simulink model "KiemnghiemDatathudc"  (R2021b)
settings: Solver=VariableStepAuto  StartTime=0.0  StopTime=10  RelTol=1e-3
InitFcn:
  | x_ref = 1; l_ref =0.2; l_ini = 0.6;
  | 
  | %ADRC' s parameter caculation
  | b0 = (ml+mc)/(mc*ml +mc*mt+ml*mt);k_ESO = 70;T_set  = 3;
  | 
  | s_cl = -5.85/T_set;
  | Kp   = s_cl^2;
  | Kd   = -2*s_cl;
  | 
  | s_ESO = k_ESO*s_cl;
  | l1        = -3*s_ESO;
  | l2        = 3*( s_ESO)^2;
  | l3        = -(s_ESO)^3;
  | 
  | %Observer
  | A = [-l1, 1, 0;
  |         -l2, 0, 1;
  |         -l3, 0, 0];
  | B = [0;
  |         b0;
  |         0];
  | L = [l1;
  |        l2;
  |        l3];
  | 
  | b1 = (mt+mc)/(mc*ml +mc*mt+ml*mt);k_ESO1 =100;T_set1  = 3;
  | s_cl1 = -5.85/T_set1;
  | Kp1   = s_cl1^2;
  | Kd1   = -2*s_cl1;
  | 
  | s_ESO1 = k_ESO1*s_cl1;
  | l11        = -3*s_ESO1;
  | l21        = 3*( s_ESO1)^2;
  | l31        = -(s_ESO1)^3;
  | 
  | %Observer
  | A1 = [-l11, 1, 0;
  |         -l21, 0, 1;
  |         -l31, 0, 0];
  | B1 = [0;
  |         b1;
  |         0];
  | L1 = [l11;
  |        l21;
  |        l31];
values from neighbouring files (symbols this model uses):
  g = 9.81    [Thong_so_double_pendulum.m]
undefined symbols (not defined in the file or in its folder): K_pso, mc, sigbuilder_block, T_pso, waof, waol
libraries: neural x95, simulink x11, simulink_extras x11
(part 2 of 6)

== system KiemnghiemDatathudc/data_l_conzvd_3neuron/Custom Neural Network ==
  Input : Inport  PortDimensions=1
      mask Display: e = 0.06;c1 = [120 230 180]/255;c2 = ([120 230 180]+0)/(256+128);c3 = ([120 230 180]+128)/(256+128);patch([0 1 1 0],[0 0 1 1],c1);patch([0 1 1 1-e 1-e 0+e],[0 0 1 1-e 0+e 0+e],c2);patch([0 0 1 1-e 0+e 0+e],[0 1 1 1-e 1-e 0+e],c3);plot([0 1 1 0 0],[0 0 1 1 0]);
  Layer 1 : Subsystem
      mask Display: e = 0.06;c1 = [120 150 230]/255;c2 = ([120 150 230]+0)/383;c3 = ([120 150 230]+128)/383;patch([0 1 1 0],[0 0 1 1],c1);patch([0 1 1 1-e 1-e 0+e],[0 0 1 1-e 0+e 0+e],c2);patch([0 0 1 1-e 0+e 0+e],[0 1 1 1-e 1-e 0+e],c3);plot([0 1 1 0 0],[0 0 1 1 0]);
  Layer 2 : Subsystem
      mask Display: e = 0.06;c1 = [120 150 230]/255;c2 = ([120 150 230]+0)/383;c3 = ([120 150 230]+128)/383;patch([0 1 1 0],[0 0 1 1],c1);patch([0 1 1 1-e 1-e 0+e],[0 0 1 1-e 0+e 0+e],c2);patch([0 0 1 1-e 0+e 0+e],[0 1 1 1-e 1-e 0+e],c3);plot([0 1 1 0 0],[0 0 1 1 0]);
  Process Input 1 : Subsystem
      mask Display: e = 0.06;c1 = [120 150 230]/255;c2 = ([120 150 230]+0)/383;c3 = ([120 150 230]+128)/383;patch([0 1 1 0],[0 0 1 1],c1);patch([0 1 1 1-e 1-e 0+e],[0 0 1 1-e 0+e 0+e],c2);patch([0 0 1 1-e 0+e 0+e],[0 1 1 1-e 1-e 0+e],c3);plot([0 1 1 0 0],[0 0 1 1 0]);
  Process Output 1 : Subsystem
      mask Display: e = 0.06;c1 = [120 150 230]/255;c2 = ([120 150 230]+0)/383;c3 = ([120 150 230]+128)/383;patch([0 1 1 0],[0 0 1 1],c1);patch([0 1 1 1-e 1-e 0+e],[0 0 1 1-e 0+e 0+e],c2);patch([0 0 1 1-e 0+e 0+e],[0 1 1 1-e 1-e 0+e],c3);plot([0 1 1 0 0],[0 0 1 1 0]);
  Output : Outport  InitialOutput=[0;0]
      mask Display: e = 0.06;c1 = [120 230 180]/255;c2 = ([120 230 180]+0)/(256+128);c3 = ([120 230 180]+128)/(256+128);patch([0 1 1 0],[0 0 1 1],c1);patch([0 1 1 1-e 1-e 0+e],[0 0 1 1-e 0+e 0+e],c2);patch([0 0 1 1-e 0+e 0+e],[0 1 1 1-e 1-e 0+e],c3);plot([0 1 1 0 0],[0 0 1 1 0]);
  wires:
  Input/1 -> Process Input 1/1(x)
  Process Output 1/1(y) -> Output/1
  Process Input 1/1(p) -> Layer 1/1("p{1}")
  Layer 1/1("a{1}") -> [feedback1]
  [feedback1] -> Layer 2/1("a{1} ")
  Layer 2/1("a{2}") -> Process Output 1/1(a)

== system KiemnghiemDatathudc/data_l_conzvd_3neuron/Fitness APS ZVD4 ==
  e : Inport
  Abs : Abs
  Abs1 : Abs
  Integrator : Integrator
  MinMax Running Resettable : simulink/Math Operations/MinMax Running Resettable  Function=max  vinit=0.0
  Step : Step  Time=0.000001  Before=1  After=0  SampleTime=0
  IAE : Outport
  MAx : Outport  Port=2
  wires:
  Abs/1 -> Integrator/1
  Abs1/1 -> MinMax Running Resettable/1
  Step/1 -> MinMax Running Resettable/2
  e/1 -> Abs/1, Abs1/1
  Integrator/1 -> IAE/1
  MinMax Running Resettable/1 -> MAx/1

== system KiemnghiemDatathudc/data_l_conzvd_3neuron/Subsystem5 ==
  ref_ZV : Inport
  ref_ZV1 : Inport  Port=2
  "ADRC " : Subsystem
  ADRC 1 : Subsystem
  Constant : Constant  Value=mc
  Gain : Gain  Gain=1/3
  Subsystem : Subsystem
  the : Outport
  x : Outport  Port=2
  l : Outport  Port=3
  wires:
  Subsystem/1(x) -> x/1, "ADRC "/2(x)  "Position"
  ADRC 1/1(u) -> Subsystem/2(ul)  "ADRC"
  Subsystem/3(the) -> Gain/1
  Subsystem/2(l) -> ADRC 1/2(x), l/1  "Length"
  "ADRC "/1(u) -> Subsystem/1(ut)  "ADRC"
  ref_ZV1/1 -> ADRC 1/1(ref)
  ref_ZV/1 -> "ADRC "/1(ref)
  Gain/1 -> the/1
  Constant/1 -> Subsystem/3(mc)

== system KiemnghiemDatathudc/data_l_conzvd_3neuron/ZVD3 ==
  ref : Inport
  Input : Inport  Port=2
  Input2 : Inport  Port=3
  Input1 : Inport  Port=4
  Gain1 : Gain  Gain=0.25
  Gain2 : Gain  Gain=0.5
  Gain3 : Gain  Gain=0.25
  MATLAB Function : MATLAB Function  TreatAsAtomicUnit=on
  MATLAB Function1 : MATLAB Function  TreatAsAtomicUnit=on
  Sum : Sum  Inputs=+++
  Variable Transport Delay : VariableTransportDelay  VariableDelayType=Variable transport delay  MaximumDelay=10
  Variable Transport Delay1 : VariableTransportDelay  VariableDelayType=Variable transport delay  MaximumDelay=10
  ref_AZ : Outport
  wires:
  Gain2/1 -> Variable Transport Delay/1
  Gain1/1 -> Sum/1
  Variable Transport Delay/1 -> Sum/2
  Sum/1 -> ref_AZ/1
  ref/1 -> Gain1/1, Gain3/1, Gain2/1
  Gain3/1 -> Variable Transport Delay1/1
  Variable Transport Delay1/1 -> Sum/3
  Input/1 -> Variable Transport Delay/2
  Input2/1 -> MATLAB Function1/1(u), MATLAB Function/1(u)
  MATLAB Function1/1(y) -> ?
  Input1/1 -> Variable Transport Delay1/2

== system KiemnghiemDatathudc/data_ml_3neuron/Custom Neural Network ==
  Input : Inport  PortDimensions=2
      mask Display: e = 0.06;c1 = [120 230 180]/255;c2 = ([120 230 180]+0)/(256+128);c3 = ([120 230 180]+128)/(256+128);patch([0 1 1 0],[0 0 1 1],c1);patch([0 1 1 1-e 1-e 0+e],[0 0 1 1-e 0+e 0+e],c2);patch([0 0 1 1-e 0+e 0+e],[0 1 1 1-e 1-e 0+e],c3);plot([0 1 1 0 0],[0 0 1 1 0]);
  Layer 1 : Subsystem
      mask Display: e = 0.06;c1 = [120 150 230]/255;c2 = ([120 150 230]+0)/383;c3 = ([120 150 230]+128)/383;patch([0 1 1 0],[0 0 1 1],c1);patch([0 1 1 1-e 1-e 0+e],[0 0 1 1-e 0+e 0+e],c2);patch([0 0 1 1-e 0+e 0+e],[0 1 1 1-e 1-e 0+e],c3);plot([0 1 1 0 0],[0 0 1 1 0]);
  Layer 2 : Subsystem
      mask Display: e = 0.06;c1 = [120 150 230]/255;c2 = ([120 150 230]+0)/383;c3 = ([120 150 230]+128)/383;patch([0 1 1 0],[0 0 1 1],c1);patch([0 1 1 1-e 1-e 0+e],[0 0 1 1-e 0+e 0+e],c2);patch([0 0 1 1-e 0+e 0+e],[0 1 1 1-e 1-e 0+e],c3);plot([0 1 1 0 0],[0 0 1 1 0]);
  Process Input 1 : Subsystem
      mask Display: e = 0.06;c1 = [120 150 230]/255;c2 = ([120 150 230]+0)/383;c3 = ([120 150 230]+128)/383;patch([0 1 1 0],[0 0 1 1],c1);patch([0 1 1 1-e 1-e 0+e],[0 0 1 1-e 0+e 0+e],c2);patch([0 0 1 1-e 0+e 0+e],[0 1 1 1-e 1-e 0+e],c3);plot([0 1 1 0 0],[0 0 1 1 0]);
  Process Output 1 : Subsystem
      mask Display: e = 0.06;c1 = [120 150 230]/255;c2 = ([120 150 230]+0)/383;c3 = ([120 150 230]+128)/383;patch([0 1 1 0],[0 0 1 1],c1);patch([0 1 1 1-e 1-e 0+e],[0 0 1 1-e 0+e 0+e],c2);patch([0 0 1 1-e 0+e 0+e],[0 1 1 1-e 1-e 0+e],c3);plot([0 1 1 0 0],[0 0 1 1 0]);
  Output : Outport  InitialOutput=[0;0]
      mask Display: e = 0.06;c1 = [120 230 180]/255;c2 = ([120 230 180]+0)/(256+128);c3 = ([120 230 180]+128)/(256+128);patch([0 1 1 0],[0 0 1 1],c1);patch([0 1 1 1-e 1-e 0+e],[0 0 1 1-e 0+e 0+e],c2);patch([0 0 1 1-e 0+e 0+e],[0 1 1 1-e 1-e 0+e],c3);plot([0 1 1 0 0],[0 0 1 1 0]);
  wires:
  Input/1 -> Process Input 1/1(x)
  Process Output 1/1(y) -> Output/1
  Process Input 1/1(p) -> Layer 1/1("p{1}")
  Layer 1/1("a{1}") -> [feedback1]
  [feedback1] -> Layer 2/1("a{1} ")
  Layer 2/1("a{2}") -> Process Output 1/1(a)

== system KiemnghiemDatathudc/data_ml_3neuron/Fitness APS ZVD4 ==
  e : Inport
  Abs : Abs
  Abs1 : Abs
  Integrator : Integrator
  MinMax Running Resettable : simulink/Math Operations/MinMax Running Resettable  Function=max  vinit=0.0
  Step : Step  Time=0.000001  Before=1  After=0  SampleTime=0
  IAE : Outport
  MAx : Outport  Port=2
  wires:
  Abs/1 -> Integrator/1
  Abs1/1 -> MinMax Running Resettable/1
  Step/1 -> MinMax Running Resettable/2
  e/1 -> Abs/1, Abs1/1
  Integrator/1 -> IAE/1
  MinMax Running Resettable/1 -> MAx/1

== system KiemnghiemDatathudc/data_ml_3neuron/Subsystem5 ==
  ref_ZV : Inport
  ref_ZV1 : Inport  Port=2
  "ADRC " : Subsystem
  ADRC 1 : Subsystem
  Constant : Constant  Value=mc
  Gain : Gain  Gain=1/3
  Subsystem : Subsystem
  the : Outport
  x : Outport  Port=2
  l : Outport  Port=3
  wires:
  Subsystem/1(x) -> x/1, "ADRC "/2(x)  "Position"
  ADRC 1/1(u) -> Subsystem/2(ul)  "ADRC"
  Subsystem/3(the) -> Gain/1
  Subsystem/2(l) -> ADRC 1/2(x), l/1  "Length"
  "ADRC "/1(u) -> Subsystem/1(ut)  "ADRC"
  ref_ZV1/1 -> ADRC 1/1(ref)
  ref_ZV/1 -> "ADRC "/1(ref)
  Gain/1 -> the/1
  Constant/1 -> Subsystem/3(mc)

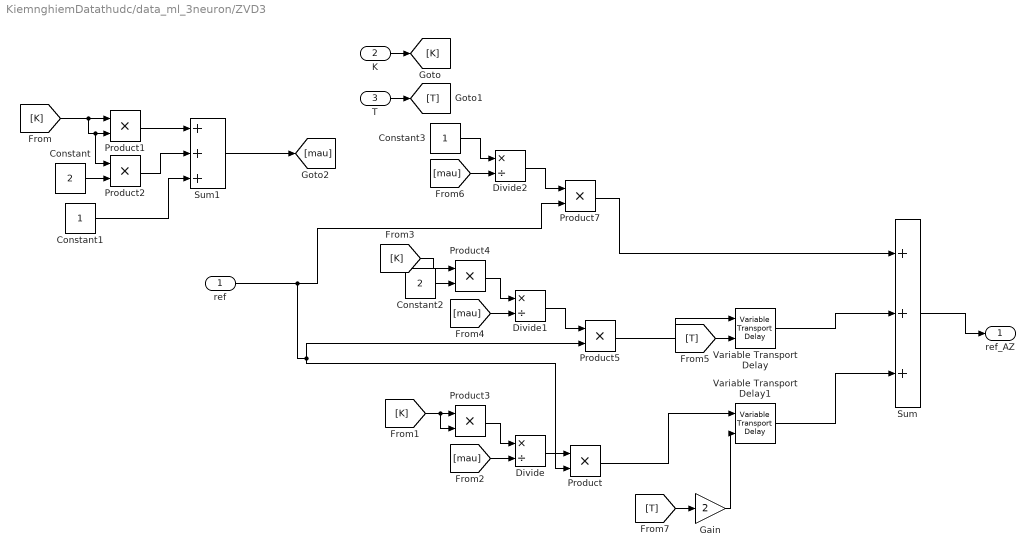
== system KiemnghiemDatathudc/data_ml_3neuron/ZVD3 ==
  ref : Inport
  K : Inport  Port=2
  T : Inport  Port=3
  Constant : Constant  Value=2
  Constant1 : Constant
  Constant2 : Constant  Value=2
  Constant3 : Constant
  Divide : Product  Inputs=*/
  Divide1 : Product  Inputs=*/
  Divide2 : Product  Inputs=*/
  Gain : Gain  Gain=2
  Product{,1..5,7} (7 alike) : Product
  Sum : Sum  Inputs=+++
  Sum1 : Sum  Inputs=+++
  Variable Transport Delay : VariableTransportDelay  VariableDelayType=Variable transport delay  MaximumDelay=10
  Variable Transport Delay1 : VariableTransportDelay  VariableDelayType=Variable transport delay  MaximumDelay=10
  ref_AZ : Outport
  wires:
  Product5/1 -> Variable Transport Delay/1
  Product7/1 -> Sum/1
  Variable Transport Delay/1 -> Sum/2
  Sum/1 -> ref_AZ/1
  ref/1 -> Product7/2, Product/2, Product5/2
  Product/1 -> Variable Transport Delay1/1
  Variable Transport Delay1/1 -> Sum/3
  K/1 -> [K]
  T/1 -> [T]
  [K] -> Product2/1, Product1/2, Product1/1
  Constant/1 -> Product2/2
  Product1/1 -> Sum1/1
  Product2/1 -> Sum1/2
  Constant1/1 -> Sum1/3
  Sum1/1 -> [mau]
  [K] -> Product4/1
  Product4/1 -> Divide1/1
  [mau] -> Divide1/2
  Divide1/1 -> Product5/1
  Constant2/1 -> Product4/2
  Constant3/1 -> Divide2/1
  Divide2/1 -> Product7/1
  [mau] -> Divide2/2
  [K] -> Product3/2, Product3/1
  Product3/1 -> Divide/1
  [mau] -> Divide/2
  Divide/1 -> Product/1
  [T] -> Variable Transport Delay/2
  [T] -> Gain/1
  Gain/1 -> Variable Transport Delay1/2

== system KiemnghiemDatathudc/data_ml_conzvd_3neuron/Custom Neural Network ==
  Input : Inport  PortDimensions=2
      mask Display: e = 0.06;c1 = [120 230 180]/255;c2 = ([120 230 180]+0)/(256+128);c3 = ([120 230 180]+128)/(256+128);patch([0 1 1 0],[0 0 1 1],c1);patch([0 1 1 1-e 1-e 0+e],[0 0 1 1-e 0+e 0+e],c2);patch([0 0 1 1-e 0+e 0+e],[0 1 1 1-e 1-e 0+e],c3);plot([0 1 1 0 0],[0 0 1 1 0]);
  Layer 1 : Subsystem
      mask Display: e = 0.06;c1 = [120 150 230]/255;c2 = ([120 150 230]+0)/383;c3 = ([120 150 230]+128)/383;patch([0 1 1 0],[0 0 1 1],c1);patch([0 1 1 1-e 1-e 0+e],[0 0 1 1-e 0+e 0+e],c2);patch([0 0 1 1-e 0+e 0+e],[0 1 1 1-e 1-e 0+e],c3);plot([0 1 1 0 0],[0 0 1 1 0]);
  Layer 2 : Subsystem
      mask Display: e = 0.06;c1 = [120 150 230]/255;c2 = ([120 150 230]+0)/383;c3 = ([120 150 230]+128)/383;patch([0 1 1 0],[0 0 1 1],c1);patch([0 1 1 1-e 1-e 0+e],[0 0 1 1-e 0+e 0+e],c2);patch([0 0 1 1-e 0+e 0+e],[0 1 1 1-e 1-e 0+e],c3);plot([0 1 1 0 0],[0 0 1 1 0]);
  Process Input 1 : Subsystem
      mask Display: e = 0.06;c1 = [120 150 230]/255;c2 = ([120 150 230]+0)/383;c3 = ([120 150 230]+128)/383;patch([0 1 1 0],[0 0 1 1],c1);patch([0 1 1 1-e 1-e 0+e],[0 0 1 1-e 0+e 0+e],c2);patch([0 0 1 1-e 0+e 0+e],[0 1 1 1-e 1-e 0+e],c3);plot([0 1 1 0 0],[0 0 1 1 0]);
  Process Output 1 : Subsystem
      mask Display: e = 0.06;c1 = [120 150 230]/255;c2 = ([120 150 230]+0)/383;c3 = ([120 150 230]+128)/383;patch([0 1 1 0],[0 0 1 1],c1);patch([0 1 1 1-e 1-e 0+e],[0 0 1 1-e 0+e 0+e],c2);patch([0 0 1 1-e 0+e 0+e],[0 1 1 1-e 1-e 0+e],c3);plot([0 1 1 0 0],[0 0 1 1 0]);
  Output : Outport  InitialOutput=[0;0]
      mask Display: e = 0.06;c1 = [120 230 180]/255;c2 = ([120 230 180]+0)/(256+128);c3 = ([120 230 180]+128)/(256+128);patch([0 1 1 0],[0 0 1 1],c1);patch([0 1 1 1-e 1-e 0+e],[0 0 1 1-e 0+e 0+e],c2);patch([0 0 1 1-e 0+e 0+e],[0 1 1 1-e 1-e 0+e],c3);plot([0 1 1 0 0],[0 0 1 1 0]);
  wires:
  Input/1 -> Process Input 1/1(x)
  Process Output 1/1(y) -> Output/1
  Process Input 1/1(p) -> Layer 1/1("p{1}")
  Layer 1/1("a{1}") -> [feedback1]
  [feedback1] -> Layer 2/1("a{1} ")
  Layer 2/1("a{2}") -> Process Output 1/1(a)

== system KiemnghiemDatathudc/data_ml_conzvd_3neuron/Fitness APS ZVD4 ==
  e : Inport
  Abs : Abs
  Abs1 : Abs
  Integrator : Integrator
  MinMax Running Resettable : simulink/Math Operations/MinMax Running Resettable  Function=max  vinit=0.0
  Step : Step  Time=0.000001  Before=1  After=0  SampleTime=0
  IAE : Outport
  MAx : Outport  Port=2
  wires:
  Abs/1 -> Integrator/1
  Abs1/1 -> MinMax Running Resettable/1
  Step/1 -> MinMax Running Resettable/2
  e/1 -> Abs/1, Abs1/1
  Integrator/1 -> IAE/1
  MinMax Running Resettable/1 -> MAx/1

== system KiemnghiemDatathudc/data_ml_conzvd_3neuron/Subsystem5 ==
  ref_ZV : Inport
  ref_ZV1 : Inport  Port=2
  "ADRC " : Subsystem
  ADRC 1 : Subsystem
  Constant : Constant  Value=mc
  Gain : Gain  Gain=1/3
  Subsystem : Subsystem
  the : Outport
  x : Outport  Port=2
  l : Outport  Port=3
  wires:
  Subsystem/1(x) -> x/1, "ADRC "/2(x)  "Position"
  ADRC 1/1(u) -> Subsystem/2(ul)  "ADRC"
  Subsystem/3(the) -> Gain/1
  Subsystem/2(l) -> ADRC 1/2(x), l/1  "Length"
  "ADRC "/1(u) -> Subsystem/1(ut)  "ADRC"
  ref_ZV1/1 -> ADRC 1/1(ref)
  ref_ZV/1 -> "ADRC "/1(ref)
  Gain/1 -> the/1
  Constant/1 -> Subsystem/3(mc)

== system KiemnghiemDatathudc/data_ml_conzvd_3neuron/ZVD3 ==
  ref : Inport
  Input : Inport  Port=2
  Input1 : Inport  Port=3
  Gain1 : Gain  Gain=0.25
  Gain2 : Gain  Gain=0.5
  Gain3 : Gain  Gain=0.25
  Sum : Sum  Inputs=+++
  Variable Transport Delay : VariableTransportDelay  VariableDelayType=Variable transport delay  MaximumDelay=10
  Variable Transport Delay1 : VariableTransportDelay  VariableDelayType=Variable transport delay  MaximumDelay=10
  ref_AZ : Outport
  wires:
  Gain2/1 -> Variable Transport Delay/1
  Gain1/1 -> Sum/1
  Variable Transport Delay/1 -> Sum/2
  Sum/1 -> ref_AZ/1
  ref/1 -> Gain1/1, Gain3/1, Gain2/1
  Gain3/1 -> Variable Transport Delay1/1
  Variable Transport Delay1/1 -> Sum/3
  Input/1 -> Variable Transport Delay/2
  Input1/1 -> Variable Transport Delay1/2

== system KiemnghiemDatathudc/net3_zvd2_3neuron/Fitness APS ZVD4 ==
  e : Inport
  Abs : Abs
  Abs1 : Abs
  Integrator : Integrator
  MinMax Running Resettable : simulink/Math Operations/MinMax Running Resettable  Function=max  vinit=0.0
  Step : Step  Time=0.000001  Before=1  After=0  SampleTime=0
  IAE : Outport
  MAx : Outport  Port=2
  wires:
  Abs/1 -> Integrator/1
  Abs1/1 -> MinMax Running Resettable/1
  Step/1 -> MinMax Running Resettable/2
  e/1 -> Abs/1, Abs1/1
  Integrator/1 -> IAE/1
  MinMax Running Resettable/1 -> MAx/1

== system KiemnghiemDatathudc/net3_zvd2_3neuron/Subsystem5 ==
  ref_ZV : Inport
  ref_ZV1 : Inport  Port=2
  "ADRC " : Subsystem
  ADRC 1 : Subsystem
  Constant : Constant  Value=mc
  Gain : Gain  Gain=1/3
  Subsystem : Subsystem
  the : Outport
  x : Outport  Port=2
  l : Outport  Port=3
  wires:
  Subsystem/1(x) -> x/1, "ADRC "/2(x)  "Position"
  ADRC 1/1(u) -> Subsystem/2(ul)  "ADRC"
  Subsystem/3(the) -> Gain/1
  Subsystem/2(l) -> ADRC 1/2(x), l/1  "Length"
  "ADRC "/1(u) -> Subsystem/1(ut)  "ADRC"
  ref_ZV1/1 -> ADRC 1/1(ref)
  ref_ZV/1 -> "ADRC "/1(ref)
  Gain/1 -> the/1
  Constant/1 -> Subsystem/3(mc)

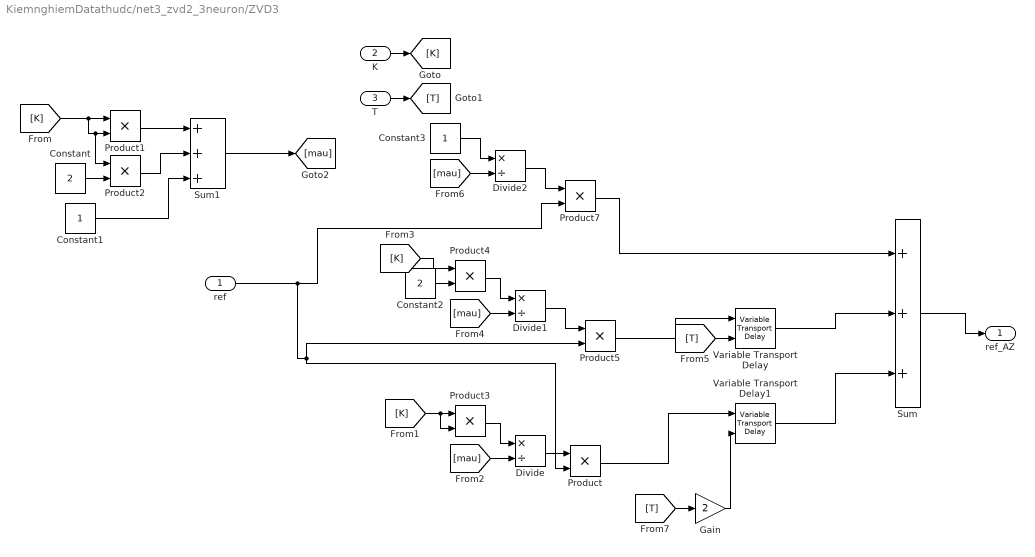
== system KiemnghiemDatathudc/net3_zvd2_3neuron/ZVD3 ==
  ref : Inport
  K : Inport  Port=2
  T : Inport  Port=3
  Constant : Constant  Value=2
  Constant1 : Constant
  Constant2 : Constant  Value=2
  Constant3 : Constant
  Divide : Product  Inputs=*/
  Divide1 : Product  Inputs=*/
  Divide2 : Product  Inputs=*/
  Gain : Gain  Gain=2
  Product{,1..5,7} (7 alike) : Product
  Sum : Sum  Inputs=+++
  Sum1 : Sum  Inputs=+++
  Variable Transport Delay : VariableTransportDelay  VariableDelayType=Variable transport delay  MaximumDelay=10
  Variable Transport Delay1 : VariableTransportDelay  VariableDelayType=Variable transport delay  MaximumDelay=10
  ref_AZ : Outport
  wires:
  Product5/1 -> Variable Transport Delay/1
  Product7/1 -> Sum/1
  Variable Transport Delay/1 -> Sum/2
  Sum/1 -> ref_AZ/1
  ref/1 -> Product7/2, Product/2, Product5/2
  Product/1 -> Variable Transport Delay1/1
  Variable Transport Delay1/1 -> Sum/3
  K/1 -> [K]
  T/1 -> [T]
  [K] -> Product2/1, Product1/2, Product1/1
  Constant/1 -> Product2/2
  Product1/1 -> Sum1/1
  Product2/1 -> Sum1/2
  Constant1/1 -> Sum1/3
  Sum1/1 -> [mau]
  [K] -> Product4/1
  Product4/1 -> Divide1/1
  [mau] -> Divide1/2
  Divide1/1 -> Product5/1
  Constant2/1 -> Product4/2
  Constant3/1 -> Divide2/1
  Divide2/1 -> Product7/1
  [mau] -> Divide2/2
  [K] -> Product3/2, Product3/1
  Product3/1 -> Divide/1
  [mau] -> Divide/2
  Divide/1 -> Product/1
  [T] -> Variable Transport Delay/2
  [T] -> Gain/1
  Gain/1 -> Variable Transport Delay1/2

== system KiemnghiemDatathudc/net3_zvd2_3neuron/net3_zvd2_3neuron ==
  Input : Inport  PortDimensions=1
      mask Display: e = 0.06;c1 = [120 230 180]/255;c2 = ([120 230 180]+0)/(256+128);c3 = ([120 230 180]+128)/(256+128);patch([0 1 1 0],[0 0 1 1],c1);patch([0 1 1 1-e 1-e 0+e],[0 0 1 1-e 0+e 0+e],c2);patch([0 0 1 1-e 0+e 0+e],[0 1 1 1-e 1-e 0+e],c3);plot([0 1 1 0 0],[0 0 1 1 0]);
  Layer 1 : Subsystem
      mask Display: e = 0.06;c1 = [120 150 230]/255;c2 = ([120 150 230]+0)/383;c3 = ([120 150 230]+128)/383;patch([0 1 1 0],[0 0 1 1],c1);patch([0 1 1 1-e 1-e 0+e],[0 0 1 1-e 0+e 0+e],c2);patch([0 0 1 1-e 0+e 0+e],[0 1 1 1-e 1-e 0+e],c3);plot([0 1 1 0 0],[0 0 1 1 0]);
  Layer 2 : Subsystem
      mask Display: e = 0.06;c1 = [120 150 230]/255;c2 = ([120 150 230]+0)/383;c3 = ([120 150 230]+128)/383;patch([0 1 1 0],[0 0 1 1],c1);patch([0 1 1 1-e 1-e 0+e],[0 0 1 1-e 0+e 0+e],c2);patch([0 0 1 1-e 0+e 0+e],[0 1 1 1-e 1-e 0+e],c3);plot([0 1 1 0 0],[0 0 1 1 0]);
  Process Input 1 : Subsystem
      mask Display: e = 0.06;c1 = [120 150 230]/255;c2 = ([120 150 230]+0)/383;c3 = ([120 150 230]+128)/383;patch([0 1 1 0],[0 0 1 1],c1);patch([0 1 1 1-e 1-e 0+e],[0 0 1 1-e 0+e 0+e],c2);patch([0 0 1 1-e 0+e 0+e],[0 1 1 1-e 1-e 0+e],c3);plot([0 1 1 0 0],[0 0 1 1 0]);
  Process Output 1 : Subsystem
      mask Display: e = 0.06;c1 = [120 150 230]/255;c2 = ([120 150 230]+0)/383;c3 = ([120 150 230]+128)/383;patch([0 1 1 0],[0 0 1 1],c1);patch([0 1 1 1-e 1-e 0+e],[0 0 1 1-e 0+e 0+e],c2);patch([0 0 1 1-e 0+e 0+e],[0 1 1 1-e 1-e 0+e],c3);plot([0 1 1 0 0],[0 0 1 1 0]);
  Output : Outport  InitialOutput=[0;0]
      mask Display: e = 0.06;c1 = [120 230 180]/255;c2 = ([120 230 180]+0)/(256+128);c3 = ([120 230 180]+128)/(256+128);patch([0 1 1 0],[0 0 1 1],c1);patch([0 1 1 1-e 1-e 0+e],[0 0 1 1-e 0+e 0+e],c2);patch([0 0 1 1-e 0+e 0+e],[0 1 1 1-e 1-e 0+e],c3);plot([0 1 1 0 0],[0 0 1 1 0]);
  wires:
  Input/1 -> Process Input 1/1(x)
  Process Output 1/1(y) -> Output/1
  Process Input 1/1(p) -> Layer 1/1("p{1}")
  Layer 1/1("a{1}") -> [feedback1]
  [feedback1] -> Layer 2/1("a{1} ")
  Layer 2/1("a{2}") -> Process Output 1/1(a)

== system KiemnghiemDatathudc/net3_zvd2_6neuron/Fitness APS ZVD4 ==
  e : Inport
  Abs : Abs
  Abs1 : Abs
  Integrator : Integrator
  MinMax Running Resettable : simulink/Math Operations/MinMax Running Resettable  Function=max  vinit=0.0
  Step : Step  Time=0.000001  Before=1  After=0  SampleTime=0
  IAE : Outport
  MAx : Outport  Port=2
  wires:
  Abs/1 -> Integrator/1
  Abs1/1 -> MinMax Running Resettable/1
  Step/1 -> MinMax Running Resettable/2
  e/1 -> Abs/1, Abs1/1
  Integrator/1 -> IAE/1
  MinMax Running Resettable/1 -> MAx/1

== system KiemnghiemDatathudc/net3_zvd2_6neuron/Subsystem5 ==
  ref_ZV : Inport
  ref_ZV1 : Inport  Port=2
  "ADRC " : Subsystem
  ADRC 1 : Subsystem
  Gain : Gain  Gain=1/3
  Subsystem : Subsystem
  the : Outport
  x : Outport  Port=2
  l : Outport  Port=3
  wires:
  Subsystem/1(x) -> x/1, "ADRC "/2(x)  "Position"
  ADRC 1/1(u) -> Subsystem/2(ul)  "ADRC"
  Subsystem/3(the) -> Gain/1
  Subsystem/2(l) -> ADRC 1/2(x), l/1  "Length"
  "ADRC "/1(u) -> Subsystem/1(ut)  "ADRC"
  ref_ZV1/1 -> ADRC 1/1(ref)
  ref_ZV/1 -> "ADRC "/1(ref)
  Gain/1 -> the/1

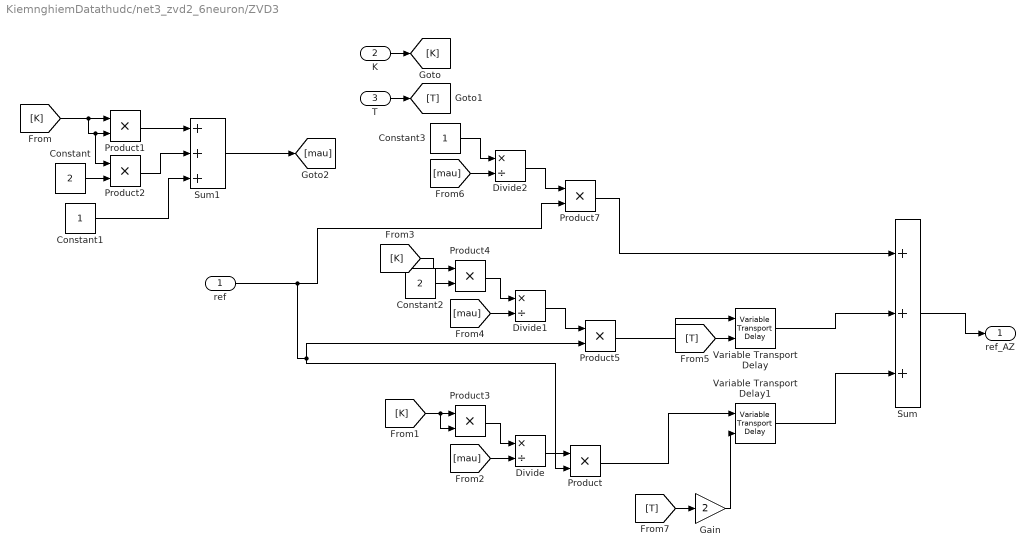
== system KiemnghiemDatathudc/net3_zvd2_6neuron/ZVD3 ==
  ref : Inport
  K : Inport  Port=2
  T : Inport  Port=3
  Constant : Constant  Value=2
  Constant1 : Constant
  Constant2 : Constant  Value=2
  Constant3 : Constant
  Divide : Product  Inputs=*/
  Divide1 : Product  Inputs=*/
  Divide2 : Product  Inputs=*/
  Gain : Gain  Gain=2
  Product{,1..5,7} (7 alike) : Product
  Sum : Sum  Inputs=+++
  Sum1 : Sum  Inputs=+++
  Variable Transport Delay : VariableTransportDelay  VariableDelayType=Variable transport delay  MaximumDelay=10
  Variable Transport Delay1 : VariableTransportDelay  VariableDelayType=Variable transport delay  MaximumDelay=10
  ref_AZ : Outport
  wires:
  Product5/1 -> Variable Transport Delay/1
  Product7/1 -> Sum/1
  Variable Transport Delay/1 -> Sum/2
  Sum/1 -> ref_AZ/1
  ref/1 -> Product7/2, Product/2, Product5/2
  Product/1 -> Variable Transport Delay1/1
  Variable Transport Delay1/1 -> Sum/3
  K/1 -> [K]
  T/1 -> [T]
  [K] -> Product2/1, Product1/2, Product1/1
  Constant/1 -> Product2/2
  Product1/1 -> Sum1/1
  Product2/1 -> Sum1/2
  Constant1/1 -> Sum1/3
  Sum1/1 -> [mau]
  [K] -> Product4/1
  Product4/1 -> Divide1/1
  [mau] -> Divide1/2
  Divide1/1 -> Product5/1
  Constant2/1 -> Product4/2
  Constant3/1 -> Divide2/1
  Divide2/1 -> Product7/1
  [mau] -> Divide2/2
  [K] -> Product3/2, Product3/1
  Product3/1 -> Divide/1
  [mau] -> Divide/2
  Divide/1 -> Product/1
  [T] -> Variable Transport Delay/2
  [T] -> Gain/1
  Gain/1 -> Variable Transport Delay1/2

== system KiemnghiemDatathudc/net3_zvd2_6neuron/net3_zvd2_6neuron ==
  Input : Inport  PortDimensions=1
      mask Display: e = 0.06;c1 = [120 230 180]/255;c2 = ([120 230 180]+0)/(256+128);c3 = ([120 230 180]+128)/(256+128);patch([0 1 1 0],[0 0 1 1],c1);patch([0 1 1 1-e 1-e 0+e],[0 0 1 1-e 0+e 0+e],c2);patch([0 0 1 1-e 0+e 0+e],[0 1 1 1-e 1-e 0+e],c3);plot([0 1 1 0 0],[0 0 1 1 0]);
  Layer 1 : Subsystem
      mask Display: e = 0.06;c1 = [120 150 230]/255;c2 = ([120 150 230]+0)/383;c3 = ([120 150 230]+128)/383;patch([0 1 1 0],[0 0 1 1],c1);patch([0 1 1 1-e 1-e 0+e],[0 0 1 1-e 0+e 0+e],c2);patch([0 0 1 1-e 0+e 0+e],[0 1 1 1-e 1-e 0+e],c3);plot([0 1 1 0 0],[0 0 1 1 0]);
  Layer 2 : Subsystem
      mask Display: e = 0.06;c1 = [120 150 230]/255;c2 = ([120 150 230]+0)/383;c3 = ([120 150 230]+128)/383;patch([0 1 1 0],[0 0 1 1],c1);patch([0 1 1 1-e 1-e 0+e],[0 0 1 1-e 0+e 0+e],c2);patch([0 0 1 1-e 0+e 0+e],[0 1 1 1-e 1-e 0+e],c3);plot([0 1 1 0 0],[0 0 1 1 0]);
  Process Input 1 : Subsystem
      mask Display: e = 0.06;c1 = [120 150 230]/255;c2 = ([120 150 230]+0)/383;c3 = ([120 150 230]+128)/383;patch([0 1 1 0],[0 0 1 1],c1);patch([0 1 1 1-e 1-e 0+e],[0 0 1 1-e 0+e 0+e],c2);patch([0 0 1 1-e 0+e 0+e],[0 1 1 1-e 1-e 0+e],c3);plot([0 1 1 0 0],[0 0 1 1 0]);
  Process Output 1 : Subsystem
      mask Display: e = 0.06;c1 = [120 150 230]/255;c2 = ([120 150 230]+0)/383;c3 = ([120 150 230]+128)/383;patch([0 1 1 0],[0 0 1 1],c1);patch([0 1 1 1-e 1-e 0+e],[0 0 1 1-e 0+e 0+e],c2);patch([0 0 1 1-e 0+e 0+e],[0 1 1 1-e 1-e 0+e],c3);plot([0 1 1 0 0],[0 0 1 1 0]);
  Output : Outport  InitialOutput=[0;0]
      mask Display: e = 0.06;c1 = [120 230 180]/255;c2 = ([120 230 180]+0)/(256+128);c3 = ([120 230 180]+128)/(256+128);patch([0 1 1 0],[0 0 1 1],c1);patch([0 1 1 1-e 1-e 0+e],[0 0 1 1-e 0+e 0+e],c2);patch([0 0 1 1-e 0+e 0+e],[0 1 1 1-e 1-e 0+e],c3);plot([0 1 1 0 0],[0 0 1 1 0]);
  wires:
  Input/1 -> Process Input 1/1(x)
  Process Output 1/1(y) -> Output/1
  Process Input 1/1(p) -> Layer 1/1("p{1}")
  Layer 1/1("a{1}") -> [feedback1]
  [feedback1] -> Layer 2/1("a{1} ")
  Layer 2/1("a{2}") -> Process Output 1/1(a)

== system KiemnghiemDatathudc/network1_3neuron/Layer 1 ==
  "p{1}" : Inport  PortDimensions=1
      mask Display: e = 0.06;c1 = [120 230 180]/255;c2 = ([120 230 180]+0)/(256+128);c3 = ([120 230 180]+128)/(256+128);patch([0 1 1 0],[0 0 1 1],c1);patch([0 1 1 1-e 1-e 0+e],[0 0 1 1-e 0+e 0+e],c2);patch([0 0 1 1-e 0+e 0+e],[0 1 1 1-e 1-e 0+e],c3);plot([0 1 1 0 0],[0 0 1 1 0]);
  Delays 1 : Subsystem
      mask Display: e = 0.06;c1 = [120 150 230]/255;c2 = ([120 150 230]+0)/383;c3 = ([120 150 230]+128)/383;patch([0 1 1 0],[0 0 1 1],c1);patch([0 1 1 1-e 1-e 0+e],[0 0 1 1-e 0+e 0+e],c2);patch([0 0 1 1-e 0+e 0+e],[0 1 1 1-e 1-e 0+e],c3);plot([0 1 1 0 0],[0 0 1 1 0]);disp('0');
  "IW{1,1}" : Subsystem
      mask Display: e = 0.06;c1 = [120 150 230]/255;c2 = ([120 150 230]+0)/383;c3 = ([120 150 230]+128)/383;patch([0 1 1 0],[0 0 1 1],c1);patch([0 1 1 1-e 1-e 0+e],[0 0 1 1-e 0+e 0+e],c2);patch([0 0 1 1-e 0+e 0+e],[0 1 1 1-e 1-e 0+e],c3);plot([0 1 1 0 0],[0 0 1 1 0]);disp('W');
  "b{1}" : Constant  Value=[8.4507777617371591105666084331460297107696533203125;5.1923231306089530079361793468706309795379638671875;-0.094564599494747714203413124778307974338531494140625]
      mask Display: e = 0.06;c1 = [120 150 230]/255;c2 = ([120 150 230]+0)/383;c3 = ([120 150 230]+128)/383;patch([0 1 1 0],[0 0 1 1],c1);patch([0 1 1 1-e 1-e 0+e],[0 0 1 1-e 0+e 0+e],c2);patch([0 0 1 1-e 0+e 0+e],[0 1 1 1-e 1-e 0+e],c3);plot([0 1 1 0 0],[0 0 1 1 0]);disp('b');
  logsig : neural/Transfer Functions/logsig
      settings: SourceProductBaseCode=NN
  netsum : Sum  Inputs=2  InputSameDT=on  SaturateOnIntegerOverflow=on  OutDataTypeStr=Inherit: Same as first input
      mask Display: e = 0.06;c1 = [120 150 230]/255;c2 = ([120 150 230]+0)/383;c3 = ([120 150 230]+128)/383;patch([0 1 1 0],[0 0 1 1],c1);patch([0 1 1 1-e 1-e 0+e],[0 0 1 1-e 0+e 0+e],c2);patch([0 0 1 1-e 0+e 0+e],[0 1 1 1-e 1-e 0+e],c3);plot([0 1 1 0 0],[0 0 1 1 0]);disp('+');
  "a{1}" : Outport  InitialOutput=[0;0;0]
      mask Display: e = 0.06;c1 = [120 230 180]/255;c2 = ([120 230 180]+0)/(256+128);c3 = ([120 230 180]+128)/(256+128);patch([0 1 1 0],[0 0 1 1],c1);patch([0 1 1 1-e 1-e 0+e],[0 0 1 1-e 0+e 0+e],c2);patch([0 0 1 1-e 0+e 0+e],[0 1 1 1-e 1-e 0+e],c3);plot([0 1 1 0 0],[0 0 1 1 0]);
  wires:
  "p{1}"/1 -> Delays 1/1("p{1}")
  Delays 1/1("pd{1,1}") -> "IW{1,1}"/1("pd{1,1}")
  "IW{1,1}"/1("iz{1,1}") -> netsum/1
  "b{1}"/1 -> netsum/2
  netsum/1 -> logsig/1
  logsig/1 -> "a{1}"/1

== system KiemnghiemDatathudc/network1_3neuron/Layer 2 ==
  "a{1} " : Inport  PortDimensions=3
      mask Display: e = 0.06;c1 = [120 230 180]/255;c2 = ([120 230 180]+0)/(256+128);c3 = ([120 230 180]+128)/(256+128);patch([0 1 1 0],[0 0 1 1],c1);patch([0 1 1 1-e 1-e 0+e],[0 0 1 1-e 0+e 0+e],c2);patch([0 0 1 1-e 0+e 0+e],[0 1 1 1-e 1-e 0+e],c3);plot([0 1 1 0 0],[0 0 1 1 0]);
  Delays 1 : Subsystem
      mask Display: e = 0.06;c1 = [120 150 230]/255;c2 = ([120 150 230]+0)/383;c3 = ([120 150 230]+128)/383;patch([0 1 1 0],[0 0 1 1],c1);patch([0 1 1 1-e 1-e 0+e],[0 0 1 1-e 0+e 0+e],c2);patch([0 0 1 1-e 0+e 0+e],[0 1 1 1-e 1-e 0+e],c3);plot([0 1 1 0 0],[0 0 1 1 0]);disp('0');
  "LW{2,1}" : Subsystem
      mask Display: e = 0.06;c1 = [120 150 230]/255;c2 = ([120 150 230]+0)/383;c3 = ([120 150 230]+128)/383;patch([0 1 1 0],[0 0 1 1],c1);patch([0 1 1 1-e 1-e 0+e],[0 0 1 1-e 0+e 0+e],c2);patch([0 0 1 1-e 0+e 0+e],[0 1 1 1-e 1-e 0+e],c3);plot([0 1 1 0 0],[0 0 1 1 0]);disp('W');
  "b{2}" : Constant  Value=[3.65574008688713636416878216550685465335845947265625;-11.009829406887774894130416214466094970703125]
      mask Display: e = 0.06;c1 = [120 150 230]/255;c2 = ([120 150 230]+0)/383;c3 = ([120 150 230]+128)/383;patch([0 1 1 0],[0 0 1 1],c1);patch([0 1 1 1-e 1-e 0+e],[0 0 1 1-e 0+e 0+e],c2);patch([0 0 1 1-e 0+e 0+e],[0 1 1 1-e 1-e 0+e],c3);plot([0 1 1 0 0],[0 0 1 1 0]);disp('b');
  logsig : neural/Transfer Functions/logsig
      settings: SourceProductBaseCode=NN
  netsum : Sum  Inputs=2  InputSameDT=on  SaturateOnIntegerOverflow=on  OutDataTypeStr=Inherit: Same as first input
      mask Display: e = 0.06;c1 = [120 150 230]/255;c2 = ([120 150 230]+0)/383;c3 = ([120 150 230]+128)/383;patch([0 1 1 0],[0 0 1 1],c1);patch([0 1 1 1-e 1-e 0+e],[0 0 1 1-e 0+e 0+e],c2);patch([0 0 1 1-e 0+e 0+e],[0 1 1 1-e 1-e 0+e],c3);plot([0 1 1 0 0],[0 0 1 1 0]);disp('+');
  "a{2}" : Outport  InitialOutput=[0;0]
      mask Display: e = 0.06;c1 = [120 230 180]/255;c2 = ([120 230 180]+0)/(256+128);c3 = ([120 230 180]+128)/(256+128);patch([0 1 1 0],[0 0 1 1],c1);patch([0 1 1 1-e 1-e 0+e],[0 0 1 1-e 0+e 0+e],c2);patch([0 0 1 1-e 0+e 0+e],[0 1 1 1-e 1-e 0+e],c3);plot([0 1 1 0 0],[0 0 1 1 0]);
  wires:
  "a{1} "/1 -> Delays 1/1("p{2}")
  Delays 1/1("pd{2,1}") -> "LW{2,1}"/1("ad{2,1}")
  "LW{2,1}"/1("lz{2,1}") -> netsum/1
  "b{2}"/1 -> netsum/2
  netsum/1 -> logsig/1
  logsig/1 -> "a{2}"/1

== system KiemnghiemDatathudc/network1_3neuron/Process Input 1 ==
  x : Inport  PortDimensions=1
      mask Display: e = 0.06;c1 = [120 230 180]/255;c2 = ([120 230 180]+0)/(256+128);c3 = ([120 230 180]+128)/(256+128);patch([0 1 1 0],[0 0 1 1],c1);patch([0 1 1 1-e 1-e 0+e],[0 0 1 1-e 0+e 0+e],c2);patch([0 0 1 1-e 0+e 0+e],[0 1 1 1-e 1-e 0+e],c3);plot([0 1 1 0 0],[0 0 1 1 0]);
  mapminmax : neural/Processing Functions/mapminmax  xmin=0.400000000000000022204460492503  xmax=0.599999999999999977795539507497  ymin=-1  ymax=1
  p : Outport  PortDimensions=1
      mask Display: e = 0.06;c1 = [120 230 180]/255;c2 = ([120 230 180]+0)/(256+128);c3 = ([120 230 180]+128)/(256+128);patch([0 1 1 0],[0 0 1 1],c1);patch([0 1 1 1-e 1-e 0+e],[0 0 1 1-e 0+e 0+e],c2);patch([0 0 1 1-e 0+e 0+e],[0 1 1 1-e 1-e 0+e],c3);plot([0 1 1 0 0],[0 0 1 1 0]);
  wires:
  x/1 -> mapminmax/1
  mapminmax/1 -> p/1

== system KiemnghiemDatathudc/network1_3neuron/Process Output 1 ==
  a : Inport  PortDimensions=2
      mask Display: e = 0.06;c1 = [120 230 180]/255;c2 = ([120 230 180]+0)/(256+128);c3 = ([120 230 180]+128)/(256+128);patch([0 1 1 0],[0 0 1 1],c1);patch([0 1 1 1-e 1-e 0+e],[0 0 1 1-e 0+e 0+e],c2);patch([0 0 1 1-e 0+e 0+e],[0 1 1 1-e 1-e 0+e],c3);plot([0 1 1 0 0],[0 0 1 1 0]);
  mapminmax_reverse : neural/Processing Functions/mapminmax_reverse  xmin=[0.954098618173775947504111627495;0.634373984921940969883280558861]  xmax=[0.995308042620397959154843192664;0.776946284577393009307400006946]  ymin=-1  ymax=1
  y : Outport  PortDimensions=2
      mask Display: e = 0.06;c1 = [120 230 180]/255;c2 = ([120 230 180]+0)/(256+128);c3 = ([120 230 180]+128)/(256+128);patch([0 1 1 0],[0 0 1 1],c1);patch([0 1 1 1-e 1-e 0+e],[0 0 1 1-e 0+e 0+e],c2);patch([0 0 1 1-e 0+e 0+e],[0 1 1 1-e 1-e 0+e],c3);plot([0 1 1 0 0],[0 0 1 1 0]);
  wires:
  a/1 -> mapminmax_reverse/1
  mapminmax_reverse/1 -> y/1

== system KiemnghiemDatathudc/network2_3neuron/Layer 1 ==
  "p{1}" : Inport  PortDimensions=1
      mask Display: e = 0.06;c1 = [120 230 180]/255;c2 = ([120 230 180]+0)/(256+128);c3 = ([120 230 180]+128)/(256+128);patch([0 1 1 0],[0 0 1 1],c1);patch([0 1 1 1-e 1-e 0+e],[0 0 1 1-e 0+e 0+e],c2);patch([0 0 1 1-e 0+e 0+e],[0 1 1 1-e 1-e 0+e],c3);plot([0 1 1 0 0],[0 0 1 1 0]);
  Delays 1 : Subsystem
      mask Display: e = 0.06;c1 = [120 150 230]/255;c2 = ([120 150 230]+0)/383;c3 = ([120 150 230]+128)/383;patch([0 1 1 0],[0 0 1 1],c1);patch([0 1 1 1-e 1-e 0+e],[0 0 1 1-e 0+e 0+e],c2);patch([0 0 1 1-e 0+e 0+e],[0 1 1 1-e 1-e 0+e],c3);plot([0 1 1 0 0],[0 0 1 1 0]);disp('0');
  "IW{1,1}" : Subsystem
      mask Display: e = 0.06;c1 = [120 150 230]/255;c2 = ([120 150 230]+0)/383;c3 = ([120 150 230]+128)/383;patch([0 1 1 0],[0 0 1 1],c1);patch([0 1 1 1-e 1-e 0+e],[0 0 1 1-e 0+e 0+e],c2);patch([0 0 1 1-e 0+e 0+e],[0 1 1 1-e 1-e 0+e],c3);plot([0 1 1 0 0],[0 0 1 1 0]);disp('W');
  "b{1}" : Constant  Value=[-12.193386380275750724422323401086032390594482421875;-1.89992944318673639969574651331640779972076416015625;-1.3294257092556513999426215377752669155597686767578125]
      mask Display: e = 0.06;c1 = [120 150 230]/255;c2 = ([120 150 230]+0)/383;c3 = ([120 150 230]+128)/383;patch([0 1 1 0],[0 0 1 1],c1);patch([0 1 1 1-e 1-e 0+e],[0 0 1 1-e 0+e 0+e],c2);patch([0 0 1 1-e 0+e 0+e],[0 1 1 1-e 1-e 0+e],c3);plot([0 1 1 0 0],[0 0 1 1 0]);disp('b');
  logsig : neural/Transfer Functions/logsig
      settings: SourceProductBaseCode=NN
  netsum : Sum  Inputs=2  InputSameDT=on  SaturateOnIntegerOverflow=on  OutDataTypeStr=Inherit: Same as first input
      mask Display: e = 0.06;c1 = [120 150 230]/255;c2 = ([120 150 230]+0)/383;c3 = ([120 150 230]+128)/383;patch([0 1 1 0],[0 0 1 1],c1);patch([0 1 1 1-e 1-e 0+e],[0 0 1 1-e 0+e 0+e],c2);patch([0 0 1 1-e 0+e 0+e],[0 1 1 1-e 1-e 0+e],c3);plot([0 1 1 0 0],[0 0 1 1 0]);disp('+');
  "a{1}" : Outport  InitialOutput=[0;0;0]
      mask Display: e = 0.06;c1 = [120 230 180]/255;c2 = ([120 230 180]+0)/(256+128);c3 = ([120 230 180]+128)/(256+128);patch([0 1 1 0],[0 0 1 1],c1);patch([0 1 1 1-e 1-e 0+e],[0 0 1 1-e 0+e 0+e],c2);patch([0 0 1 1-e 0+e 0+e],[0 1 1 1-e 1-e 0+e],c3);plot([0 1 1 0 0],[0 0 1 1 0]);
  wires:
  "p{1}"/1 -> Delays 1/1("p{1}")
  Delays 1/1("pd{1,1}") -> "IW{1,1}"/1("pd{1,1}")
  "IW{1,1}"/1("iz{1,1}") -> netsum/1
  "b{1}"/1 -> netsum/2
  netsum/1 -> logsig/1
  logsig/1 -> "a{1}"/1

== system KiemnghiemDatathudc/network2_3neuron/Layer 2 ==
  "a{1} " : Inport  PortDimensions=3
      mask Display: e = 0.06;c1 = [120 230 180]/255;c2 = ([120 230 180]+0)/(256+128);c3 = ([120 230 180]+128)/(256+128);patch([0 1 1 0],[0 0 1 1],c1);patch([0 1 1 1-e 1-e 0+e],[0 0 1 1-e 0+e 0+e],c2);patch([0 0 1 1-e 0+e 0+e],[0 1 1 1-e 1-e 0+e],c3);plot([0 1 1 0 0],[0 0 1 1 0]);
  Delays 1 : Subsystem
      mask Display: e = 0.06;c1 = [120 150 230]/255;c2 = ([120 150 230]+0)/383;c3 = ([120 150 230]+128)/383;patch([0 1 1 0],[0 0 1 1],c1);patch([0 1 1 1-e 1-e 0+e],[0 0 1 1-e 0+e 0+e],c2);patch([0 0 1 1-e 0+e 0+e],[0 1 1 1-e 1-e 0+e],c3);plot([0 1 1 0 0],[0 0 1 1 0]);disp('0');
  "LW{2,1}" : Subsystem
      mask Display: e = 0.06;c1 = [120 150 230]/255;c2 = ([120 150 230]+0)/383;c3 = ([120 150 230]+128)/383;patch([0 1 1 0],[0 0 1 1],c1);patch([0 1 1 1-e 1-e 0+e],[0 0 1 1-e 0+e 0+e],c2);patch([0 0 1 1-e 0+e 0+e],[0 1 1 1-e 1-e 0+e],c3);plot([0 1 1 0 0],[0 0 1 1 0]);disp('W');
  "b{2}" : Constant  Value=[-8.07284681356392042061997926793992519378662109375;-3.371812931760349574261681482312269508838653564453125]
      mask Display: e = 0.06;c1 = [120 150 230]/255;c2 = ([120 150 230]+0)/383;c3 = ([120 150 230]+128)/383;patch([0 1 1 0],[0 0 1 1],c1);patch([0 1 1 1-e 1-e 0+e],[0 0 1 1-e 0+e 0+e],c2);patch([0 0 1 1-e 0+e 0+e],[0 1 1 1-e 1-e 0+e],c3);plot([0 1 1 0 0],[0 0 1 1 0]);disp('b');
  logsig : neural/Transfer Functions/logsig
      settings: SourceProductBaseCode=NN
  netsum : Sum  Inputs=2  InputSameDT=on  SaturateOnIntegerOverflow=on  OutDataTypeStr=Inherit: Same as first input
      mask Display: e = 0.06;c1 = [120 150 230]/255;c2 = ([120 150 230]+0)/383;c3 = ([120 150 230]+128)/383;patch([0 1 1 0],[0 0 1 1],c1);patch([0 1 1 1-e 1-e 0+e],[0 0 1 1-e 0+e 0+e],c2);patch([0 0 1 1-e 0+e 0+e],[0 1 1 1-e 1-e 0+e],c3);plot([0 1 1 0 0],[0 0 1 1 0]);disp('+');
  "a{2}" : Outport  InitialOutput=[0;0]
      mask Display: e = 0.06;c1 = [120 230 180]/255;c2 = ([120 230 180]+0)/(256+128);c3 = ([120 230 180]+128)/(256+128);patch([0 1 1 0],[0 0 1 1],c1);patch([0 1 1 1-e 1-e 0+e],[0 0 1 1-e 0+e 0+e],c2);patch([0 0 1 1-e 0+e 0+e],[0 1 1 1-e 1-e 0+e],c3);plot([0 1 1 0 0],[0 0 1 1 0]);
  wires:
  "a{1} "/1 -> Delays 1/1("p{2}")
  Delays 1/1("pd{2,1}") -> "LW{2,1}"/1("ad{2,1}")
  "LW{2,1}"/1("lz{2,1}") -> netsum/1
  "b{2}"/1 -> netsum/2
  netsum/1 -> logsig/1
  logsig/1 -> "a{2}"/1

== system KiemnghiemDatathudc/network2_3neuron/Process Input 1 ==
  x : Inport  PortDimensions=1
      mask Display: e = 0.06;c1 = [120 230 180]/255;c2 = ([120 230 180]+0)/(256+128);c3 = ([120 230 180]+128)/(256+128);patch([0 1 1 0],[0 0 1 1],c1);patch([0 1 1 1-e 1-e 0+e],[0 0 1 1-e 0+e 0+e],c2);patch([0 0 1 1-e 0+e 0+e],[0 1 1 1-e 1-e 0+e],c3);plot([0 1 1 0 0],[0 0 1 1 0]);
  mapminmax : neural/Processing Functions/mapminmax  xmin=0.400000000000000022204460492503  xmax=0.599999999999999977795539507497  ymin=-1  ymax=1
  p : Outport  PortDimensions=1
      mask Display: e = 0.06;c1 = [120 230 180]/255;c2 = ([120 230 180]+0)/(256+128);c3 = ([120 230 180]+128)/(256+128);patch([0 1 1 0],[0 0 1 1],c1);patch([0 1 1 1-e 1-e 0+e],[0 0 1 1-e 0+e 0+e],c2);patch([0 0 1 1-e 0+e 0+e],[0 1 1 1-e 1-e 0+e],c3);plot([0 1 1 0 0],[0 0 1 1 0]);
  wires:
  x/1 -> mapminmax/1
  mapminmax/1 -> p/1

== system KiemnghiemDatathudc/network2_3neuron/Process Output 1 ==
  a : Inport  PortDimensions=2
      mask Display: e = 0.06;c1 = [120 230 180]/255;c2 = ([120 230 180]+0)/(256+128);c3 = ([120 230 180]+128)/(256+128);patch([0 1 1 0],[0 0 1 1],c1);patch([0 1 1 1-e 1-e 0+e],[0 0 1 1-e 0+e 0+e],c2);patch([0 0 1 1-e 0+e 0+e],[0 1 1 1-e 1-e 0+e],c3);plot([0 1 1 0 0],[0 0 1 1 0]);
  mapminmax_reverse : neural/Processing Functions/mapminmax_reverse  xmin=[0.954191653406704975992624895298;0.634373984921940969883280558861]  xmax=[0.995931324853393973306481257168;0.776946284577393009307400006946]  ymin=-1  ymax=1
  y : Outport  PortDimensions=2
      mask Display: e = 0.06;c1 = [120 230 180]/255;c2 = ([120 230 180]+0)/(256+128);c3 = ([120 230 180]+128)/(256+128);patch([0 1 1 0],[0 0 1 1],c1);patch([0 1 1 1-e 1-e 0+e],[0 0 1 1-e 0+e 0+e],c2);patch([0 0 1 1-e 0+e 0+e],[0 1 1 1-e 1-e 0+e],c3);plot([0 1 1 0 0],[0 0 1 1 0]);
  wires:
  a/1 -> mapminmax_reverse/1
  mapminmax_reverse/1 -> y/1

== system KiemnghiemDatathudc/network2_6neuron/Fitness APS ZVD4 ==
  e : Inport
  Abs : Abs
  Abs1 : Abs
  Integrator : Integrator
  MinMax Running Resettable : simulink/Math Operations/MinMax Running Resettable  Function=max  vinit=0.0
  Step : Step  Time=0.000001  Before=1  After=0  SampleTime=0
  IAE : Outport
  MAx : Outport  Port=2
  wires:
  Abs/1 -> Integrator/1
  Abs1/1 -> MinMax Running Resettable/1
  Step/1 -> MinMax Running Resettable/2
  e/1 -> Abs/1, Abs1/1
  Integrator/1 -> IAE/1
  MinMax Running Resettable/1 -> MAx/1

== system KiemnghiemDatathudc/network2_6neuron/Subsystem5 ==
  ref_ZV : Inport
  ref_ZV1 : Inport  Port=2
  "ADRC " : Subsystem
  ADRC 1 : Subsystem
  Gain : Gain  Gain=1/3
  Subsystem : Subsystem
  the : Outport
  x : Outport  Port=2
  l : Outport  Port=3
  wires:
  Subsystem/1(x) -> x/1, "ADRC "/2(x)  "Position"
  ADRC 1/1(u) -> Subsystem/2(ul)  "ADRC"
  Subsystem/3(the) -> Gain/1
  Subsystem/2(l) -> ADRC 1/2(x), l/1  "Length"
  "ADRC "/1(u) -> Subsystem/1(ut)  "ADRC"
  ref_ZV1/1 -> ADRC 1/1(ref)
  ref_ZV/1 -> "ADRC "/1(ref)
  Gain/1 -> the/1

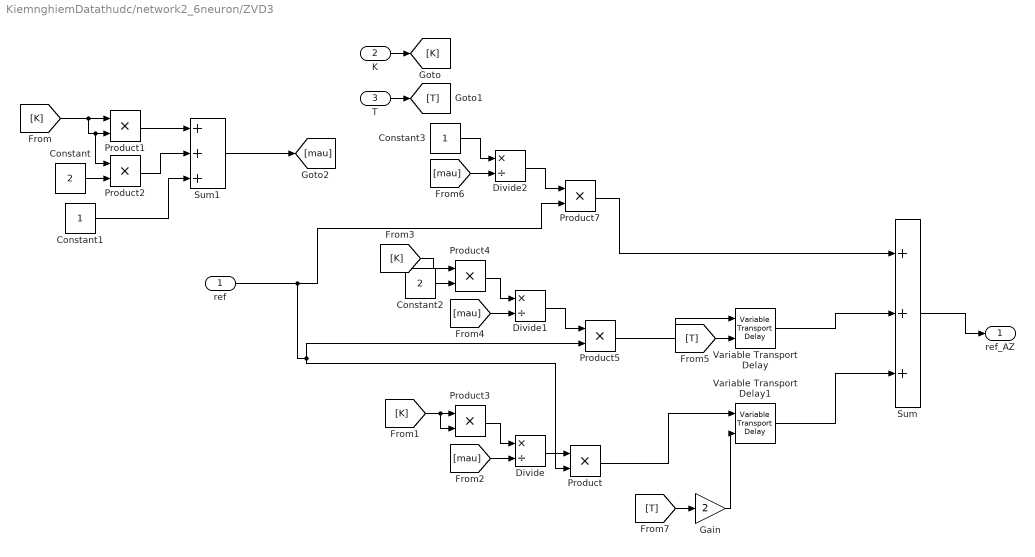
== system KiemnghiemDatathudc/network2_6neuron/ZVD3 ==
  ref : Inport
  K : Inport  Port=2
  T : Inport  Port=3
  Constant : Constant  Value=2
  Constant1 : Constant
  Constant2 : Constant  Value=2
  Constant3 : Constant
  Divide : Product  Inputs=*/
  Divide1 : Product  Inputs=*/
  Divide2 : Product  Inputs=*/
  Gain : Gain  Gain=2
  Product{,1..5,7} (7 alike) : Product
  Sum : Sum  Inputs=+++
  Sum1 : Sum  Inputs=+++
  Variable Transport Delay : VariableTransportDelay  VariableDelayType=Variable transport delay  MaximumDelay=10
  Variable Transport Delay1 : VariableTransportDelay  VariableDelayType=Variable transport delay  MaximumDelay=10
  ref_AZ : Outport
  wires:
  Product5/1 -> Variable Transport Delay/1
  Product7/1 -> Sum/1
  Variable Transport Delay/1 -> Sum/2
  Sum/1 -> ref_AZ/1
  ref/1 -> Product7/2, Product/2, Product5/2
  Product/1 -> Variable Transport Delay1/1
  Variable Transport Delay1/1 -> Sum/3
  K/1 -> [K]
  T/1 -> [T]
  [K] -> Product2/1, Product1/2, Product1/1
  Constant/1 -> Product2/2
  Product1/1 -> Sum1/1
  Product2/1 -> Sum1/2
  Constant1/1 -> Sum1/3
  Sum1/1 -> [mau]
  [K] -> Product4/1
  Product4/1 -> Divide1/1
  [mau] -> Divide1/2
  Divide1/1 -> Product5/1
  Constant2/1 -> Product4/2
  Constant3/1 -> Divide2/1
  Divide2/1 -> Product7/1
  [mau] -> Divide2/2
  [K] -> Product3/2, Product3/1
  Product3/1 -> Divide/1
  [mau] -> Divide/2
  Divide/1 -> Product/1
  [T] -> Variable Transport Delay/2
  [T] -> Gain/1
  Gain/1 -> Variable Transport Delay1/2

== system KiemnghiemDatathudc/network2_6neuron/network2_6neuron ==
  Input : Inport  PortDimensions=1
      mask Display: e = 0.06;c1 = [120 230 180]/255;c2 = ([120 230 180]+0)/(256+128);c3 = ([120 230 180]+128)/(256+128);patch([0 1 1 0],[0 0 1 1],c1);patch([0 1 1 1-e 1-e 0+e],[0 0 1 1-e 0+e 0+e],c2);patch([0 0 1 1-e 0+e 0+e],[0 1 1 1-e 1-e 0+e],c3);plot([0 1 1 0 0],[0 0 1 1 0]);
  Layer 1 : Subsystem
      mask Display: e = 0.06;c1 = [120 150 230]/255;c2 = ([120 150 230]+0)/383;c3 = ([120 150 230]+128)/383;patch([0 1 1 0],[0 0 1 1],c1);patch([0 1 1 1-e 1-e 0+e],[0 0 1 1-e 0+e 0+e],c2);patch([0 0 1 1-e 0+e 0+e],[0 1 1 1-e 1-e 0+e],c3);plot([0 1 1 0 0],[0 0 1 1 0]);
  Layer 2 : Subsystem
      mask Display: e = 0.06;c1 = [120 150 230]/255;c2 = ([120 150 230]+0)/383;c3 = ([120 150 230]+128)/383;patch([0 1 1 0],[0 0 1 1],c1);patch([0 1 1 1-e 1-e 0+e],[0 0 1 1-e 0+e 0+e],c2);patch([0 0 1 1-e 0+e 0+e],[0 1 1 1-e 1-e 0+e],c3);plot([0 1 1 0 0],[0 0 1 1 0]);
  Process Input 1 : Subsystem
      mask Display: e = 0.06;c1 = [120 150 230]/255;c2 = ([120 150 230]+0)/383;c3 = ([120 150 230]+128)/383;patch([0 1 1 0],[0 0 1 1],c1);patch([0 1 1 1-e 1-e 0+e],[0 0 1 1-e 0+e 0+e],c2);patch([0 0 1 1-e 0+e 0+e],[0 1 1 1-e 1-e 0+e],c3);plot([0 1 1 0 0],[0 0 1 1 0]);
  Process Output 1 : Subsystem
      mask Display: e = 0.06;c1 = [120 150 230]/255;c2 = ([120 150 230]+0)/383;c3 = ([120 150 230]+128)/383;patch([0 1 1 0],[0 0 1 1],c1);patch([0 1 1 1-e 1-e 0+e],[0 0 1 1-e 0+e 0+e],c2);patch([0 0 1 1-e 0+e 0+e],[0 1 1 1-e 1-e 0+e],c3);plot([0 1 1 0 0],[0 0 1 1 0]);
  Output : Outport  InitialOutput=[0;0]
      mask Display: e = 0.06;c1 = [120 230 180]/255;c2 = ([120 230 180]+0)/(256+128);c3 = ([120 230 180]+128)/(256+128);patch([0 1 1 0],[0 0 1 1],c1);patch([0 1 1 1-e 1-e 0+e],[0 0 1 1-e 0+e 0+e],c2);patch([0 0 1 1-e 0+e 0+e],[0 1 1 1-e 1-e 0+e],c3);plot([0 1 1 0 0],[0 0 1 1 0]);
  wires:
  Input/1 -> Process Input 1/1(x)
  Process Output 1/1(y) -> Output/1
  Process Input 1/1(p) -> Layer 1/1("p{1}")
  Layer 1/1("a{1}") -> [feedback1]
  [feedback1] -> Layer 2/1("a{1} ")
  Layer 2/1("a{2}") -> Process Output 1/1(a)

== system KiemnghiemDatathudc/ANN1/Layer 1/Delays 1 ==
  "p{1}" : Inport  PortDimensions=1
      mask Display: e = 0.06;c1 = [120 230 180]/255;c2 = ([120 230 180]+0)/(256+128);c3 = ([120 230 180]+128)/(256+128);patch([0 1 1 0],[0 0 1 1],c1);patch([0 1 1 1-e 1-e 0+e],[0 0 1 1-e 0+e 0+e],c2);patch([0 0 1 1-e 0+e 0+e],[0 1 1 1-e 1-e 0+e],c3);plot([0 1 1 0 0],[0 0 1 1 0]);
  mux : Mux  Inputs=1
      mask Display: e = 0.06;c1 = [120 150 230]/255;c2 = ([120 150 230]+0)/383;c3 = ([120 150 230]+128)/383;patch([0 1 1 0],[0 0 1 1],c1);patch([0 1 1 1-e 1-e 0+e],[0 0 1 1-e 0+e 0+e],c2);patch([0 0 1 1-e 0+e 0+e],[0 1 1 1-e 1-e 0+e],c3);plot([0 1 1 0 0],[0 0 1 1 0]);disp('Mux')
  "pd{1,1}" : Outport
      mask Display: e = 0.06;c1 = [120 230 180]/255;c2 = ([120 230 180]+0)/(256+128);c3 = ([120 230 180]+128)/(256+128);patch([0 1 1 0],[0 0 1 1],c1);patch([0 1 1 1-e 1-e 0+e],[0 0 1 1-e 0+e 0+e],c2);patch([0 0 1 1-e 0+e 0+e],[0 1 1 1-e 1-e 0+e],c3);plot([0 1 1 0 0],[0 0 1 1 0]);
  wires:
  "p{1}"/1 -> mux/1
  mux/1 -> "pd{1,1}"/1

== system KiemnghiemDatathudc/ANN1/Layer 1/IW{1,1} ==
  "pd{1,1}" : Inport  PortDimensions=1
      mask Display: e = 0.06;c1 = [120 230 180]/255;c2 = ([120 230 180]+0)/(256+128);c3 = ([120 230 180]+128)/(256+128);patch([0 1 1 0],[0 0 1 1],c1);patch([0 1 1 1-e 1-e 0+e],[0 0 1 1-e 0+e 0+e],c2);patch([0 0 1 1-e 0+e 0+e],[0 1 1 1-e 1-e 0+e],c3);plot([0 1 1 0 0],[0 0 1 1 0]);
  "IW{1,1}(1,:)'" : Constant  Value=2.880567021006085415280040251673199236392974853515625
      mask Display: e = 0.06;c1 = [120 150 230]/255;c2 = ([120 150 230]+0)/383;c3 = ([120 150 230]+128)/383;patch([0 1 1 0],[0 0 1 1],c1);patch([0 1 1 1-e 1-e 0+e],[0 0 1 1-e 0+e 0+e],c2);patch([0 0 1 1-e 0+e 0+e],[0 1 1 1-e 1-e 0+e],c3);plot([0 1 1 0 0],[0 0 1 1 0]);disp('Weights');
  "IW{1,1}(2,:)'" : Constant  Value=-2.762154438657994592887234830413945019245147705078125
      mask Display: e = 0.06;c1 = [120 150 230]/255;c2 = ([120 150 230]+0)/383;c3 = ([120 150 230]+128)/383;patch([0 1 1 0],[0 0 1 1],c1);patch([0 1 1 1-e 1-e 0+e],[0 0 1 1-e 0+e 0+e],c2);patch([0 0 1 1-e 0+e 0+e],[0 1 1 1-e 1-e 0+e],c3);plot([0 1 1 0 0],[0 0 1 1 0]);disp('Weights');
  "IW{1,1}(3,:)'" : Constant  Value=4.48929135846372862062025888008065521717071533203125
      mask Display: e = 0.06;c1 = [120 150 230]/255;c2 = ([120 150 230]+0)/383;c3 = ([120 150 230]+128)/383;patch([0 1 1 0],[0 0 1 1],c1);patch([0 1 1 1-e 1-e 0+e],[0 0 1 1-e 0+e 0+e],c2);patch([0 0 1 1-e 0+e 0+e],[0 1 1 1-e 1-e 0+e],c3);plot([0 1 1 0 0],[0 0 1 1 0]);disp('Weights');
  Mux : Mux  Inputs=3
      mask Display: e = 0.06;c1 = [120 150 230]/255;c2 = ([120 150 230]+0)/383;c3 = ([120 150 230]+128)/383;patch([0 1 1 0],[0 0 1 1],c1);patch([0 1 1 1-e 1-e 0+e],[0 0 1 1-e 0+e 0+e],c2);patch([0 0 1 1-e 0+e 0+e],[0 1 1 1-e 1-e 0+e],c3);plot([0 1 1 0 0],[0 0 1 1 0]);disp('Mux');
  dotprod1 : neural/Weight Functions/dotprod
  dotprod2 : neural/Weight Functions/dotprod
  dotprod3 : neural/Weight Functions/dotprod
  "iz{1,1}" : Outport
      mask Display: e = 0.06;c1 = [120 230 180]/255;c2 = ([120 230 180]+0)/(256+128);c3 = ([120 230 180]+128)/(256+128);patch([0 1 1 0],[0 0 1 1],c1);patch([0 1 1 1-e 1-e 0+e],[0 0 1 1-e 0+e 0+e],c2);patch([0 0 1 1-e 0+e 0+e],[0 1 1 1-e 1-e 0+e],c3);plot([0 1 1 0 0],[0 0 1 1 0]);
  wires:
  "IW{1,1}(1,:)'"/1 -> dotprod1/1
  "pd{1,1}"/1 -> dotprod1/2, dotprod2/2, dotprod3/2
  dotprod1/1 -> Mux/1
  "IW{1,1}(2,:)'"/1 -> dotprod2/1
  dotprod2/1 -> Mux/2
  "IW{1,1}(3,:)'"/1 -> dotprod3/1
  dotprod3/1 -> Mux/3
  Mux/1 -> "iz{1,1}"/1

== system KiemnghiemDatathudc/ANN1/Layer 2/Delays 1 ==
  "p{2}" : Inport  PortDimensions=3
      mask Display: e = 0.06;c1 = [120 230 180]/255;c2 = ([120 230 180]+0)/(256+128);c3 = ([120 230 180]+128)/(256+128);patch([0 1 1 0],[0 0 1 1],c1);patch([0 1 1 1-e 1-e 0+e],[0 0 1 1-e 0+e 0+e],c2);patch([0 0 1 1-e 0+e 0+e],[0 1 1 1-e 1-e 0+e],c3);plot([0 1 1 0 0],[0 0 1 1 0]);
  mux : Mux  Inputs=1
      mask Display: e = 0.06;c1 = [120 150 230]/255;c2 = ([120 150 230]+0)/383;c3 = ([120 150 230]+128)/383;patch([0 1 1 0],[0 0 1 1],c1);patch([0 1 1 1-e 1-e 0+e],[0 0 1 1-e 0+e 0+e],c2);patch([0 0 1 1-e 0+e 0+e],[0 1 1 1-e 1-e 0+e],c3);plot([0 1 1 0 0],[0 0 1 1 0]);disp('Mux')
  "pd{2,1}" : Outport
      mask Display: e = 0.06;c1 = [120 230 180]/255;c2 = ([120 230 180]+0)/(256+128);c3 = ([120 230 180]+128)/(256+128);patch([0 1 1 0],[0 0 1 1],c1);patch([0 1 1 1-e 1-e 0+e],[0 0 1 1-e 0+e 0+e],c2);patch([0 0 1 1-e 0+e 0+e],[0 1 1 1-e 1-e 0+e],c3);plot([0 1 1 0 0],[0 0 1 1 0]);
  wires:
  "p{2}"/1 -> mux/1
  mux/1 -> "pd{2,1}"/1

== system KiemnghiemDatathudc/ANN1/Layer 2/LW{2,1} ==
  "ad{2,1}" : Inport  PortDimensions=3
      mask Display: e = 0.06;c1 = [120 230 180]/255;c2 = ([120 230 180]+0)/(256+128);c3 = ([120 230 180]+128)/(256+128);patch([0 1 1 0],[0 0 1 1],c1);patch([0 1 1 1-e 1-e 0+e],[0 0 1 1-e 0+e 0+e],c2);patch([0 0 1 1-e 0+e 0+e],[0 1 1 1-e 1-e 0+e],c3);plot([0 1 1 0 0],[0 0 1 1 0]);
  "IW{2,1}(1,:)'" : Constant  Value=[-0.0708526909409556149288533788421773351728916168212890625;0.462096584209399974252363563209655694663524627685546875;-0.57211295598406353146714309332310222089290618896484375]
      mask Display: e = 0.06;c1 = [120 150 230]/255;c2 = ([120 150 230]+0)/383;c3 = ([120 150 230]+128)/383;patch([0 1 1 0],[0 0 1 1],c1);patch([0 1 1 1-e 1-e 0+e],[0 0 1 1-e 0+e 0+e],c2);patch([0 0 1 1-e 0+e 0+e],[0 1 1 1-e 1-e 0+e],c3);plot([0 1 1 0 0],[0 0 1 1 0]);disp('weights');
  "IW{2,1}(2,:)'" : Constant  Value=[0.0726131511941498219986357298694201745092868804931640625;-0.37038561711407236298754241943242959678173065185546875;-0.27229446063409035172497851817752234637737274169921875]
      mask Display: e = 0.06;c1 = [120 150 230]/255;c2 = ([120 150 230]+0)/383;c3 = ([120 150 230]+128)/383;patch([0 1 1 0],[0 0 1 1],c1);patch([0 1 1 1-e 1-e 0+e],[0 0 1 1-e 0+e 0+e],c2);patch([0 0 1 1-e 0+e 0+e],[0 1 1 1-e 1-e 0+e],c3);plot([0 1 1 0 0],[0 0 1 1 0]);disp('weights');
  Mux : Mux  Inputs=2
      mask Display: e = 0.06;c1 = [120 150 230]/255;c2 = ([120 150 230]+0)/383;c3 = ([120 150 230]+128)/383;patch([0 1 1 0],[0 0 1 1],c1);patch([0 1 1 1-e 1-e 0+e],[0 0 1 1-e 0+e 0+e],c2);patch([0 0 1 1-e 0+e 0+e],[0 1 1 1-e 1-e 0+e],c3);plot([0 1 1 0 0],[0 0 1 1 0]);disp('Mux');
  dotprod1 : neural/Weight Functions/dotprod
  dotprod2 : neural/Weight Functions/dotprod
  "lz{2,1}" : Outport
      mask Display: e = 0.06;c1 = [120 230 180]/255;c2 = ([120 230 180]+0)/(256+128);c3 = ([120 230 180]+128)/(256+128);patch([0 1 1 0],[0 0 1 1],c1);patch([0 1 1 1-e 1-e 0+e],[0 0 1 1-e 0+e 0+e],c2);patch([0 0 1 1-e 0+e 0+e],[0 1 1 1-e 1-e 0+e],c3);plot([0 1 1 0 0],[0 0 1 1 0]);
  wires:
  "IW{2,1}(1,:)'"/1 -> dotprod1/1
  "ad{2,1}"/1 -> dotprod1/2, dotprod2/2
  dotprod1/1 -> Mux/1
  "IW{2,1}(2,:)'"/1 -> dotprod2/1
  dotprod2/1 -> Mux/2
  Mux/1 -> "lz{2,1}"/1

== system KiemnghiemDatathudc/AOL/Subsystem5/ADRC  ==
  ref : Inport
  x : Inport  Port=2
  Gain : Gain  Gain=Kp
  Gain1 : Gain  Gain=Kd
  Gain2 : Gain  Gain=1/b0
  Observer : Subsystem
  Sum : Sum  Inputs=|+-
  Sum3 : Sum  Inputs=|+-
  Sum4 : Sum  Inputs=|+-
  u : Outport
  wires:
  Sum4/1 -> Gain2/1
  Sum/1 -> Gain/1
  Gain2/1 -> u/1, Observer/1(u)
  x/1 -> Observer/2(x)
  Sum3/1 -> Sum4/1
  Observer/2(x2) -> Gain1/1
  Gain1/1 -> Sum3/2
  Gain/1 -> Sum3/1
  ref/1 -> Sum/1
  Observer/1(x3) -> Sum4/2
  Observer/3(x1) -> Sum/2
